simulink model "parte1_eje16_controlAA"  (R2017b)
settings: Solver=VariableStepAuto  StartTime=0.0  StopTime=10.0  RelTol=1e-3
settings Model: Creator=cjuar  LastModifiedBy=cjuar

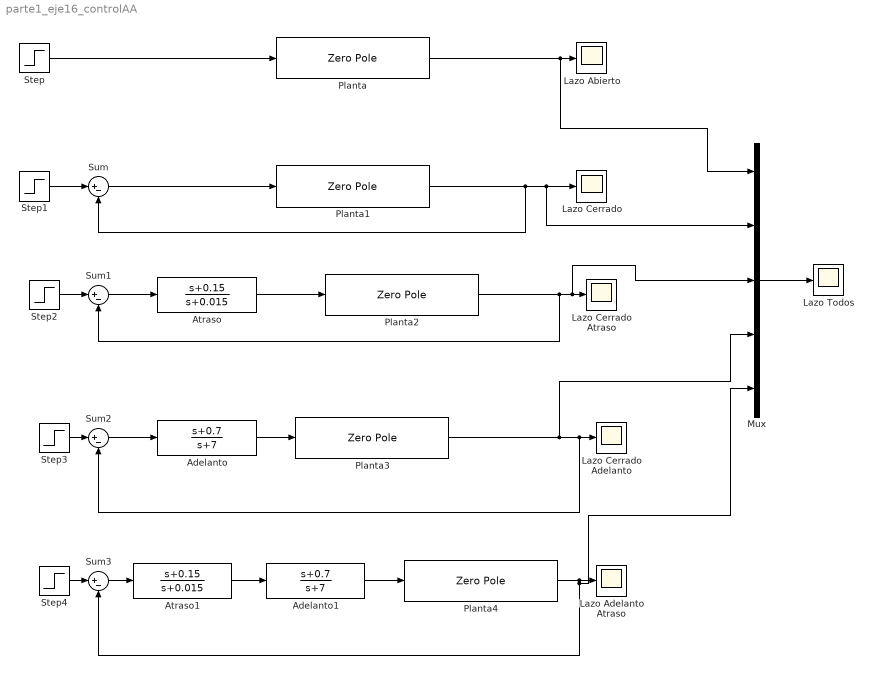
== system parte1_eje16_controlAA ==
  Adelanto : TransferFcn  Numerator=[1 0.7]  Denominator=[1 7]
  Adelanto1 : TransferFcn  Numerator=[1 0.7]  Denominator=[1 7]
  Atraso : TransferFcn  Numerator=[1 0.15]  Denominator=[1 0.015]
  Atraso1 : TransferFcn  Numerator=[1 0.15]  Denominator=[1 0.015]
  Lazo Abierto : Scope
  Lazo Adelanto Atraso : Scope
  Lazo Cerrado : Scope
  Lazo Cerrado Adelanto : Scope
  Lazo Cerrado Atraso : Scope
  Lazo Todos : Scope
  Mux : Mux  Inputs=5
  Planta{,1..4} (5 alike) : ZeroPole  Zeros=[]  Poles=[0 -1 -2]  Gain=[20]
  Step{,1..4} (5 alike) : Step  SampleTime=0
  Sum{,1..3} (4 alike) : Sum  Inputs=|+-
  wires:
  Step/1 -> Planta/1
  Planta/1 -> Mux/1, Lazo Abierto/1
  Planta1/1 -> Sum/2, Mux/2, Lazo Cerrado/1
  Step1/1 -> Sum/1
  Planta2/1 -> Sum1/2, Mux/3, Lazo Cerrado Atraso/1
  Planta3/1 -> Mux/4, Sum2/2, Lazo Cerrado Adelanto/1
  Sum/1 -> Planta1/1
  Atraso/1 -> Planta2/1
  Adelanto/1 -> Planta3/1
  Step2/1 -> Sum1/1
  Sum1/1 -> Atraso/1
  Step3/1 -> Sum2/1
  Sum2/1 -> Adelanto/1
  Sum3/1 -> Atraso1/1
  Planta4/1 -> Mux/5, Sum3/2, Lazo Adelanto Atraso/1
  Atraso1/1 -> Adelanto1/1
  Step4/1 -> Sum3/1
  Adelanto1/1 -> Planta4/1
  Mux/1 -> Lazo Todos/1
